simulink model "spring_simulator"  (R2024a)
settings: Solver=FixedStepAuto  StartTime=0.0  StopTime=50  FixedStep=0.01  RelTol=1e-3
values from neighbouring files (symbols this model uses):
  beta = 2    [params.m]
  g = 9.81    [params.m]
  initial_L = 0    [params.m]
  initial_theta = 0.5    [params.m]
  k = 10    [params.m]
  L0 = 1.0    (= 1)    [params.m]
  m = 1.0    (= 1)    [params.m]
settings Model: Creator=lucid  LastModifiedBy=lucid

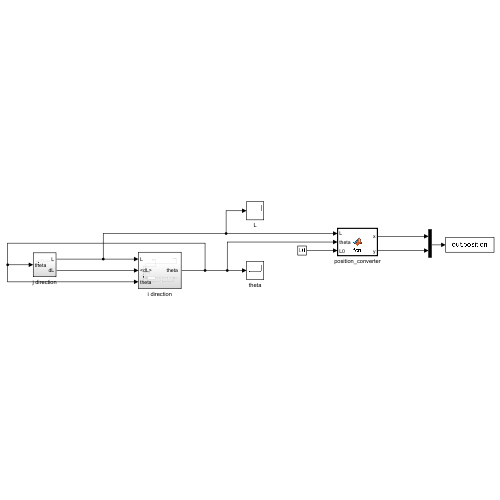
[thumbnail: Simulink's stored preview of the top-level diagram]
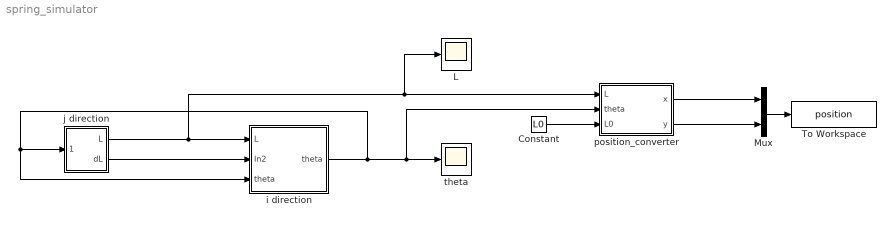
== system spring_simulator ==
  Constant : Constant  Value=L0
  L : Scope
  Mux : Mux  Inputs=2
  To Workspace : ToWorkspace  VariableName=position  SaveFormat=Structure With Time  SampleTime=-1
  i direction : Subsystem
  j direction : Subsystem
  position_converter : MATLAB Function  TreatAsAtomicUnit=on
  theta : Scope
  wires:
  j direction/1(L) -> i direction/1(L), L/1, position_converter/1(L)
  i direction/1("theta ") -> j direction/1(theta), i direction/3(theta), position_converter/2(theta), theta/1
  j direction/2(dL) -> i direction/2(In2)
  Constant/1 -> position_converter/3(L0)
  position_converter/1(x) -> Mux/1
  position_converter/2(y) -> Mux/2
  Mux/1 -> To Workspace/1

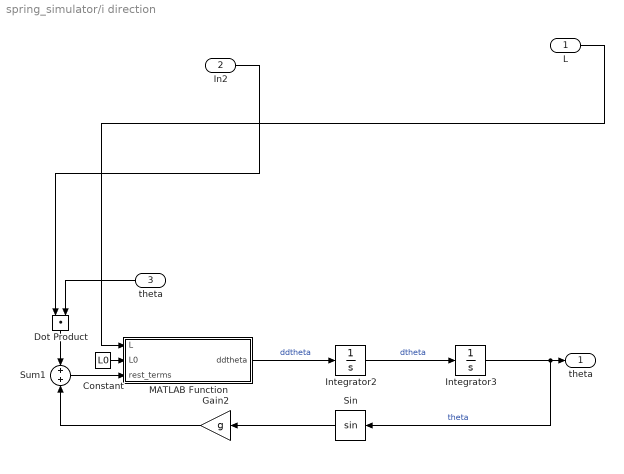
== system spring_simulator/i direction ==
  L : Inport
  In2 : Inport  Port=2
  theta : Inport  Port=3
  Constant : Constant  Value=L0
  Dot Product : DotProduct  OutDataTypeStr=Inherit: Inherit via internal rule
  Gain2 : Gain  Gain=g
  Integrator2 : Integrator
  Integrator3 : Integrator  InitialCondition=initial_theta
  MATLAB Function : MATLAB Function  TreatAsAtomicUnit=on
  Sin : Trigonometry
  Sum1 : Sum  Inputs=+|+
  "theta " : Outport
  wires:
  Gain2/1 -> Sum1/2
  Sin/1 -> Gain2/1
  Integrator3/1 -> Sin/1, "theta "/1  "theta"
  MATLAB Function/1(ddtheta) -> Integrator2/1  "ddtheta"
  Dot Product/1 -> Sum1/1
  L/1 -> MATLAB Function/1(L)
  Constant/1 -> MATLAB Function/2(L0)
  Integrator2/1 -> Integrator3/1  "dtheta"
  Sum1/1 -> MATLAB Function/3(rest_terms)
  theta/1 -> Dot Product/2
  In2/1 -> Dot Product/1

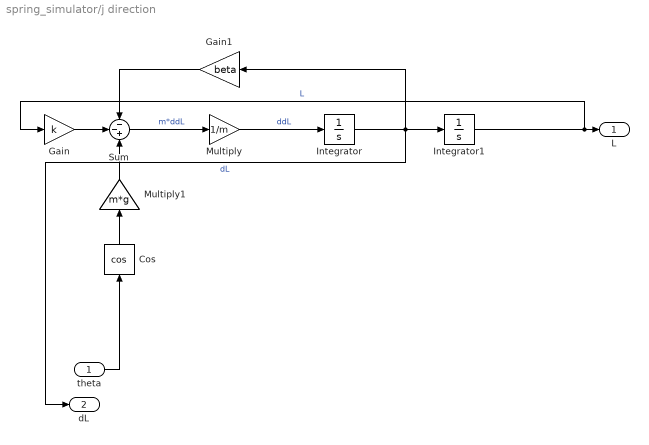
== system spring_simulator/j direction ==
  theta : Inport
  Cos : Trigonometry  Operator=cos
  Gain : Gain  Gain=k
  Gain1 : Gain  Gain=beta
  Integrator : Integrator
  Integrator1 : Integrator  InitialCondition=initial_L
  Multiply : Gain  Gain=1/m
  Multiply1 : Gain  Gain=m*g
  Sum : Sum  Inputs=--+
  L : Outport
  dL : Outport  Port=2
  wires:
  Integrator/1 -> dL/1, Gain1/1, Integrator1/1  "dL"
  Sum/1 -> Multiply/1  "m*ddL"
  Gain1/1 -> Sum/1
  Multiply/1 -> Integrator/1  "ddL"
  Cos/1 -> Multiply1/1
  Multiply1/1 -> Sum/3
  Gain/1 -> Sum/2
  theta/1 -> Cos/1
  Integrator1/1 -> Gain/1, L/1  "L"

== matlab function spring_simulator/position_converter ==
  data: x output; L input; y output; theta input; L0 input
function [x, y]= fcn(L, theta, L0)

x = (L + L0) * sin(theta);

y = - (L + L0) * cos(theta);

== matlab function spring_simulator/i direction/MATLAB Function ==
  data: L input; L0 input; rest_terms input; ddtheta output
function ddtheta = fcn(L, L0, rest_terms)

ddtheta = - rest_terms / (L + L0);
